simulink model "DCmotor"  (R2020b)
settings: Solver=VariableStepAuto  StartTime=0.0  StopTime=10.0  RelTol=1e-3
settings Model: Creator=celal  LastModifiedBy=celal

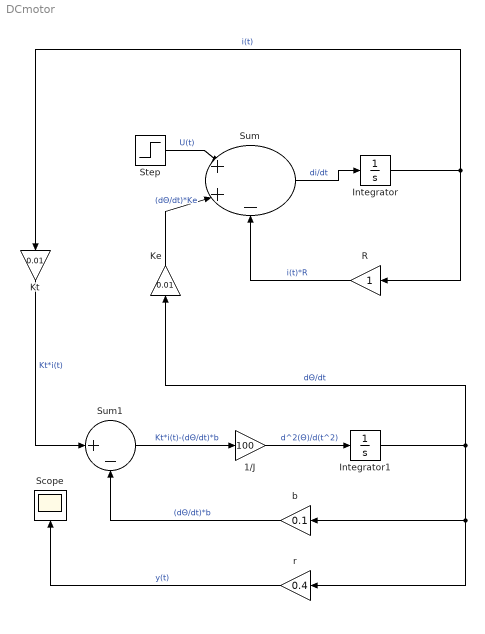
== system DCmotor ==
  1/J : Gain  Gain=100
  Integrator : Integrator
  Integrator1 : Integrator
  Ke : Gain  Gain=0.01
  Kt : Gain  Gain=0.01
  R : Gain
  Scope : Scope
  Step : Step  SampleTime=0
  Sum : Sum  Inputs=|++-
  Sum1 : Sum  Inputs=|+-
  b : Gain  Gain=0.1
  r : Gain  Gain=0.4
  wires:
  Integrator/1 -> R/1, Kt/1  "i(t)"
  Sum/1 -> Integrator/1  "di/dt"
  R/1 -> Sum/3  "i(t)*R"
  1/J/1 -> Integrator1/1  "d^2(Θ)/d(t^2)"
  Integrator1/1 -> r/1, b/1, Ke/1  "dΘ/dt"
  Ke/1 -> Sum/2  "(dΘ/dt)*Ke"
  Step/1 -> Sum/1  "U(t)"
  Sum1/1 -> 1/J/1  "Kt*i(t)-(dΘ/dt)*b"
  b/1 -> Sum1/2  "(dΘ/dt)*b"
  Kt/1 -> Sum1/1  "Kt*i(t)"
  r/1 -> Scope/1  "y(t)"
